simulink subsystem "BatteryMappedSSC"  (R2023a)
settings: Solver=VariableStepAuto  StartTime=0.0  StopTime=10.0  RelTol=1e-3
undefined symbols (not defined in the file): Bat, PlntBattChrgMax, PlntBattIntrnRes, PlntBattNumCellPar, PlntBattNumCellSer, PlntBattOpenCirctVolt, PlntBattSocBpt, PlntBattTempBpt, PlntBattVoltSocBpt
libraries: fl_lib x7, nesl_utility_internal x4, batteryecm_lib x1, nesl_utility x1
settings Model: ModifiedByFormat=The MathWorks, Inc.  Creator=The MathWorks, Inc.  LastModifiedBy=The MathWorks, Inc.
settings OptimizationCC: ReuseModelBlockBuffer=off

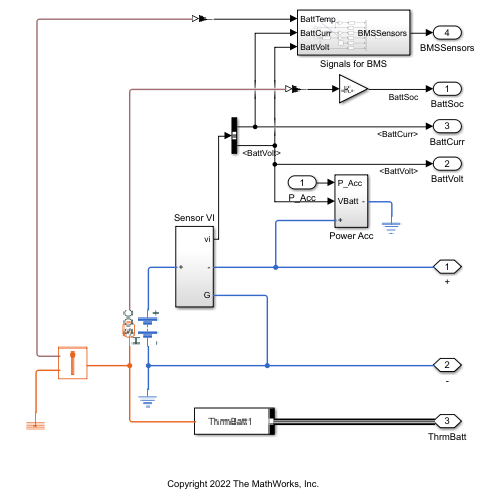
[thumbnail: Simulink's stored preview of the top-level diagram]
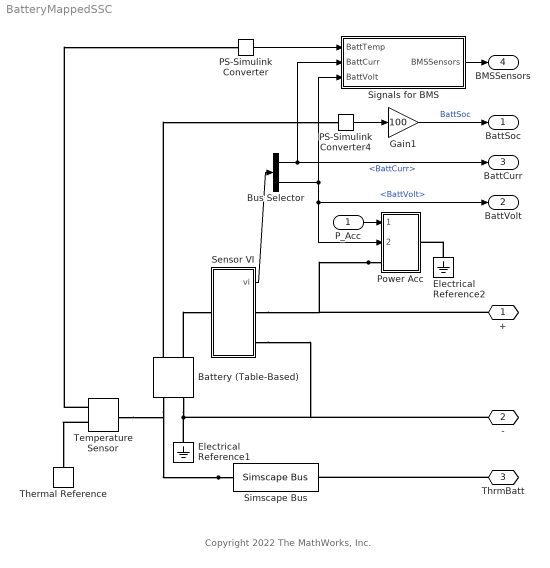
== system BatteryMappedSSC ==
  note: Copyright 2022 The MathWorks, Inc.
  P_Acc : Inport
  Battery (Table-Based) : batteryecm_lib/Battery (Table-Based)  SOC_vec=PlntBattSocBpt  T_dependence=simscape.enum.tablebattery.temperature_dependence.yes  prm_dir=simscape.enum.tablebattery.prm_dir.noCurrentDirectionality  T_vec=PlntBattTempBpt K  V0_mat=repmat(interp1(PlntBattVoltSocBpt, PlntBattOpenCirctVolt, PlntBattSocBpt)', 1, length(PlntBattTempBpt)).*PlntBattNumCellSer V  V0_vec=[3.5057, 3.566, 3.6337, 3.7127, 3.9259, 4.0777, 4.1928] V  V_range=[min(PlntBattOpenCirctVolt), inf].*PlntBattNumCellSer V  R0_mat=PlntBattIntrnRes'.*(PlntBattNumCellSer/PlntBattNumCellPar) Ohm  R0_vec=[.0085, .0085, .0087, .0082, .0083, .0085, .0085] Ohm  R0_dis_mat=[.0117, .0085, .009; .011, .0085, .009; .0114, .0087, .0092; .0107, .0082, .0088; .0107, .0083, .0091; .0113, .0085, .0089; .0116, .0085, .0089] Ohm  R0_dis_vec=[.0085, .0085, .0087, .0082, .0083, .0085, .0085] Ohm  R0_ch_mat=[.0117, .0085, .009; .011, .0085, .009; .0114, .0087, .0092; .0107, .0082, .0088; .0107, .0083, .0091; .0113, .0085, .0089; .0116, .0085, .0089] Ohm  R0_ch_vec=[.0085, .0085, .0087, .0082, .0083, .0085, .0085] Ohm  AH=PlntBattChrgMax*PlntBattNumCellPar A*hr  prm_leak=simscape.enum.tablebattery.prm_leak.disabled  Rleak_vec=[8000, 7000, 6000] Ohm  Rleak=7e3 Ohm  extrapolation_option=simscape.enum.extrapolation.nearest  SOC_port=simscape.enum.tablebattery.enable.yes  prm_dyn=simscape.enum.tablebattery.prm_dyn.off  R1_mat=[.0109, .0029, .0013; .0069, .0024, .0012; .0047, .0026, .0013; .0034, .0016, .001; .0033, .0023, .0014; .0033, .0018, .0011; .0028, .0017, .0011] Ohm  R1_vec=[.0029, .0024, .0026, .0016, .0023, .0018, .0017] Ohm  tau1_mat=[20, 36, 39; 31, 45, 39; 109, 105, 61; 36, 29, 26; 59, 77, 67; 40, 33, 29; 25, 39, 33] s  tau1_vec=[36, 45, 105, 29, 77, 33, 39] s  R2_mat=[.0109, .0029, .0013; .0069, .0024, .0012; .0047, .0026, .0013; .0034, .0016, .001; .0033, .0023, .0014; .0033, .0018, .0011; .0028, .0017, .0011] Ohm  R2_vec=[.0029, .0024, .0026, .0016, .0023, .0018, .0017] Ohm  tau2_mat=[20, 36, 39; 31, 45, 39; 109, 105, 61; 36, 29, 26; 59, 77, 67; 40, 33, 29; 25, 39, 33] s  tau2_vec=[36, 45, 105, 29, 77, 33, 39] s  R3_mat=[.0109, .0029, .0013; .0069, .0024, .0012; .0047, .0026, .0013; .0034, .0016, .001; .0033, .0023, .0014; .0033, .0018, .0011; .0028, .0017, .0011] Ohm  R3_vec=[.0029, .0024, .0026, .0016, .0023, .0018, .0017] Ohm  tau3_mat=[20, 36, 39; 31, 45, 39; 109, 105, 61; 36, 29, 26; 59, 77, 67; 40, 33, 29; 25, 39, 33] s  tau3_vec=[36, 45, 105, 29, 77, 33, 39] s  R4_mat=[.0109, .0029, .0013; .0069, .0024, .0012; .0047, .0026, .0013; .0034, .0016, .001; .0033, .0023, .0014; .0033, .0018, .0011; .0028, .0017, .0011] Ohm  R4_vec=[.0029, .0024, .0026, .0016, .0023, .0018, .0017] Ohm  tau4_mat=[20, 36, 39; 31, 45, 39; 109, 105, 61; 36, 29, 26; 59, 77, 67; 40, 33, 29; 25, 39, 33] s  tau4_vec=[36, 45, 105, 29, 77, 33, 39] s  R5_mat=[.0109, .0029, .0013; .0069, .0024, .0012; .0047, .0026, .0013; .0034, .0016, .001; .0033, .0023, .0014; .0033, .0018, .0011; .0028, .0017, .0011] Ohm  R5_vec=[.0029, .0024, .0026, .0016, .0023, .0018, .0017] Ohm  tau5_mat=[20, 36, 39; 31, 45, 39; 109, 105, 61; 36, 29, 26; 59, 77, 67; 40, 33, 29; 25, 39, 33] s  tau5_vec=[36, 45, 105, 29, 77, 33, 39] s  prm_fade=simscape.enum.tablebattery.prm_fade.disabled  N0=100  dV0=0  dR0=0  dAH=0  dRleak=0  dR1=0  dR2=0  dR3=0  dR4=0  dR5=0  N0vec=[100, 200, 300]  Tfadevec=[298.15, 323.15] K  dV0vec=[0, 0, 0]  dR0vec=[0, 0, 0]  dAHvec=[0, 0, 0]  dRleakvec=[0, 0, 0]  dR1vec=[0, 0, 0]  dR2vec=[0, 0, 0]  dR3vec=[0, 0, 0]  dR4vec=[0, 0, 0]  dR5vec=[0, 0, 0]  dV0mat=[0, 0; 0, 0; 0, 0]  dR0mat=[0, 0; 0, 0; 0, 0]  dAHmat=[0, 0; 0, 0; 0, 0]  dRleakmat=[0, 0; 0, 0; 0, 0]  dR1mat=[0, 0; 0, 0; 0, 0]  dR2mat=[0, 0; 0, 0; 0, 0]  dR3mat=[0, 0; 0, 0; 0, 0]  dR4mat=[0, 0; 0, 0; 0, 0]  dR5mat=[0, 0; 0, 0; 0, 0]  prm_age_modeling=simscape.enum.tablebattery.prm_age_modeling.equation  storage_dt_age_vec=[0] d  storage_T_age_vec=[273] K  prm_age_OCV=simscape.enum.tablebattery.prm_age_OCV.OCV  OCV_age=0.9  SOC_age=0.6  prm_age_resistance=simscape.enum.tablebattery.prm_age.disabled  OCV_scaling_age_resistance=2.2134e6  OCV_offset_age_resistance=1.632e6  temp_exp_age_resistance=0.515833569 V  t_exp_age_resistance=0.75  T_age_vec_resistance=[273.15, 298.15, 323.15] K  dt_age_vec_resistance=[90, 180, 270, 360] d  dR0_age_vec=[0, 0, 0]  t_meas_dR0_age=100 d  dR0_age_mat=[0, 0, 0; 0, 0, 0; 0, 0, 0; 0, 0, 0]  prm_age_capacity=simscape.enum.tablebattery.prm_age.disabled  OCV_scaling_age_capacity=1.5097e07  OCV_offset_age_capacity=8.3625e06  temp_exp_age_capacity=0.6011 V  t_exp_age_capacity=0.75  T_age_vec_capacity=[273.15, 298.15, 323.15] K  dt_age_vec_capacity=[90, 180, 270, 360] d  dAH_age_vec=[0, 0, 0]  t_meas_dAH_age=100 d  dAH_age_mat=[0, 0, 0; 0, 0, 0; 0, 0, 0; 0, 0, 0]  thermal_port=simscape.enum.thermaleffects.model  temperature=298.15 K  thermal_mass=PlntDCDCThermMass*PlntBattNumCellSer*PlntBattModNumCellPar % Parameter assumed J/K  i_specify=off  i_priority=None  i=0 A  i_nominal_specify=off  i_nominal_unit=A  i_nominal_value=1  v_specify=off  v_priority=None  v=0 V  v_nominal_specify=off  v_nominal_unit=V  v_nominal_value=1  stateOfCharge_specify=on  stateOfCharge_priority=High  stateOfCharge=PlntBattSocInit  stateOfCharge_nominal_specify=off  stateOfCharge_nominal_unit=1  stateOfCharge_nominal_value=1  num_cycles_specify=off  num_cycles_priority=High  num_cycles=0  num_cycles_nominal_specify=off  num_cycles_nominal_unit=1  num_cycles_nominal_value=1  cell_temperature_specify=on  cell_temperature_priority=High  cell_temperature=PlntBattTempInitDegC degC  cell_temperature_nominal_specify=off  cell_temperature_nominal_unit=K  cell_temperature_nominal_value=1
  Bus Selector : BusSelector  OutputSignals=BattCurr,BattVolt
  Electrical Reference1 : fl_lib/Electrical/Electrical Elements/Electrical Reference
  Electrical Reference2 : fl_lib/Electrical/Electrical Elements/Electrical Reference
  Gain1 : Gain  Gain=100
  PS-Simulink Converter : nesl_utility/PS-Simulink Converter  PhysicalDomain=network_engine_domain  SubClassName=ps_output  LeftPortType=input  RightPortType=output  PseudoPeriodic=off  Frequencies=[]  VectorFormat=inherit  Unit=inherit  AffineConversion=off
  PS-Simulink Converter4 : nesl_utility_internal/PS-Simulink Converter  PhysicalDomain=network_engine_domain  SubClassName=ps_output  LeftPortType=input  RightPortType=output  PseudoPeriodic=off  Frequencies=[]  VectorFormat=1-D array  Unit=1  AffineConversion=off
  Power Acc : Subsystem
  Sensor VI : Subsystem
  Signals for BMS : Subsystem
  Simscape Bus : SimscapeBus  HierarchyStrings=ThrmBatt1
  Temperature Sensor : fl_lib/Thermal/Thermal Sensors/Temperature Sensor  temperature_measure=foundation.enum.MeasurementReference.difference
  Thermal Reference : fl_lib/Thermal/Thermal Elements/Thermal Reference
  + : PMIOPort  Side=Right
  - : PMIOPort  Port=2  Side=Right
  ThrmBatt : PMIOPort  Port=3  Side=Right
  BattSoc : Outport
  BattVolt : Outport  Port=2
  BattCurr : Outport  Port=3
  BMSSensors : Outport  Port=4  VectorParamsAs1DForOutWhenUnconnected=off
  wires:
  PS-Simulink Converter4/1 -> Gain1/1
  Bus Selector/1 -> Signals for BMS/2(BattCurr), BattCurr/1  "<BattCurr>"
  Sensor VI/1(vi) -> Bus Selector/1
  Gain1/1 -> BattSoc/1  "BattSoc"
  Bus Selector/2 -> Signals for BMS/3(BattVolt), Power Acc/2(VBatt), BattVolt/1  "<BattVolt>"
  P_Acc/1 -> Power Acc/1(P_Acc)
  Signals for BMS/1(BMSSensors) -> BMSSensors/1
  PS-Simulink Converter/1 -> Signals for BMS/1(BattTemp)
  connections:
  Battery (Table-Based)/RConn1 -- Sensor VI/RConn2 -- -/RConn1 -- Electrical Reference1/LConn1
  Power Acc/LConn1 -- Sensor VI/RConn1 -- +/RConn1
  Simscape Bus/LConn1 -- Temperature Sensor/LConn1 -- Battery (Table-Based)/RConn2
  Battery (Table-Based)/LConn1 -- Sensor VI/LConn1
  Electrical Reference2/LConn1 -- Power Acc/RConn1
  Battery (Table-Based)/LConn2 -- PS-Simulink Converter4/LConn1
  Temperature Sensor/RConn1 -- Thermal Reference/LConn1
  Temperature Sensor/RConn2 -- PS-Simulink Converter/LConn1
  ThrmBatt/RConn1 -- Simscape Bus/RConn1

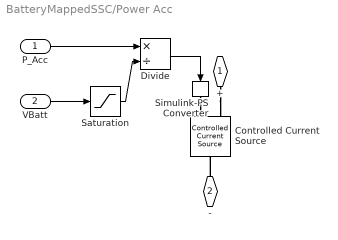
== system BatteryMappedSSC/Power Acc ==
  P_Acc : Inport
  VBatt : Inport  Port=2
  Controlled Current Source : fl_lib/Electrical/Electrical Sources/Controlled Current Source
  Divide : Product  Inputs=*/
  Saturation : Saturate  UpperLimit=inf  LowerLimit=min(Bat.noLoadV, [], 'all')  ZeroCross=off
  Simulink-PS Converter : nesl_utility_internal/Simulink-PS Converter  PhysicalDomain=network_engine_domain  SubClassName=ps_input  LeftPortType=input  RightPortType=output  PseudoPeriodic=off  Frequencies=[]  NoiseDistribution=none  NoiseParameters=[]  Unit=A  AffineConversion=off  FilteringAndDerivatives=filter  SimscapeFilterOrder=1  InputFilterTimeConstant=0.001  UdotUserProvided=0
  + : PMIOPort  Side=Left
  - : PMIOPort  Port=2  Side=Right
  wires:
  VBatt/1 -> Saturation/1
  P_Acc/1 -> Divide/1
  Divide/1 -> Simulink-PS Converter/1
  Saturation/1 -> Divide/2
  connections:
  -/RConn1 -- Controlled Current Source/LConn1
  +/RConn1 -- Controlled Current Source/RConn2
  Simulink-PS Converter/RConn1 -- Controlled Current Source/RConn1

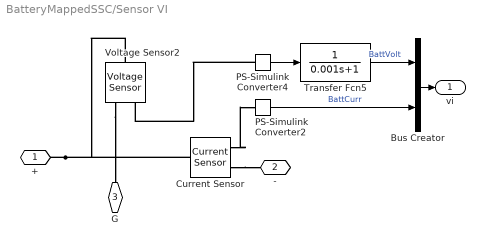
== system BatteryMappedSSC/Sensor VI ==
  Bus Creator : BusCreator  Inputs=2
  Current Sensor : fl_lib/Electrical/Electrical Sensors/Current Sensor
  PS-Simulink Converter2 : nesl_utility_internal/PS-Simulink Converter  PhysicalDomain=network_engine_domain  SubClassName=ps_output  LeftPortType=input  RightPortType=output  PseudoPeriodic=off  Frequencies=[]  VectorFormat=1-D array  Unit=1  AffineConversion=off
  PS-Simulink Converter4 : nesl_utility_internal/PS-Simulink Converter  PhysicalDomain=network_engine_domain  SubClassName=ps_output  LeftPortType=input  RightPortType=output  PseudoPeriodic=off  Frequencies=[]  VectorFormat=1-D array  Unit=1  AffineConversion=off
  Transfer Fcn5 : TransferFcn  Denominator=[0.001 1]
  Voltage Sensor2 : fl_lib/Electrical/Electrical Sensors/Voltage Sensor
  + : PMIOPort  Side=Left
  - : PMIOPort  Port=2  Side=Right
  G : PMIOPort  Port=3  Side=Right
  vi : Outport
  wires:
  Transfer Fcn5/1 -> Bus Creator/1  "BattVolt"
  PS-Simulink Converter2/1 -> Bus Creator/2  "BattCurr"
  PS-Simulink Converter4/1 -> Transfer Fcn5/1
  Bus Creator/1 -> vi/1
  connections:
  +/RConn1 -- Current Sensor/LConn1 -- Voltage Sensor2/LConn1
  PS-Simulink Converter4/LConn1 -- Voltage Sensor2/RConn1
  Current Sensor/RConn2 -- -/RConn1
  Voltage Sensor2/RConn2 -- G/RConn1
  Current Sensor/RConn1 -- PS-Simulink Converter2/LConn1

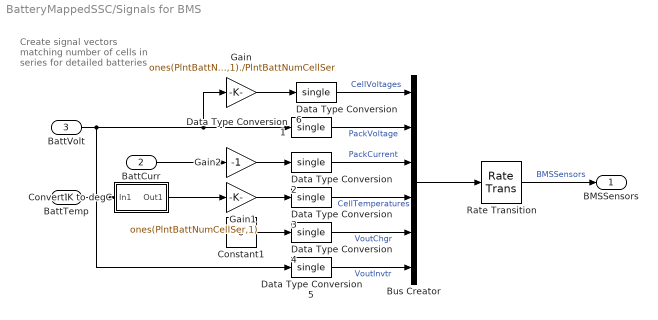
== system BatteryMappedSSC/Signals for BMS ==
  note: Create signal vectors
      | matching number of
      | cells in series for
      | detailed batteries
  BattTemp : Inport
  BattCurr : Inport  Port=2
  BattVolt : Inport  Port=3
  Bus Creator : BusCreator  Inputs=6
  Constant1 : Constant  Value=0
  Convert K to degC : Subsystem
  Data Type Conversion{1..6} (6 alike) : DataTypeConversion  OutDataTypeStr=single  SaturateOnIntegerOverflow=off  RndMeth=Floor
  Gain : Gain  Gain=ones(PlntBattNumCellSer,1)./PlntBattNumCellSer
  Gain1 : Gain  Gain=ones(PlntBattNumCellSer,1)
  Gain2 : Gain  Gain=-1
  Rate Transition : RateTransition  OutPortSampleTime=0.1
  BMSSensors : Outport
  wires:
  BattCurr/1 -> Gain2/1
  Constant1/1 -> Data Type Conversion4/1
  BattVolt/1 -> Data Type Conversion1/1, Gain/1, Data Type Conversion5/1
  Gain/1 -> Data Type Conversion6/1
  BattTemp/1 -> Convert K to degC/1(In1)
  Data Type Conversion4/1 -> Bus Creator/5  "VoutChgr"
  Gain1/1 -> Data Type Conversion3/1
  Data Type Conversion5/1 -> Bus Creator/6  "VoutInvtr"
  Gain2/1 -> Data Type Conversion2/1
  Convert K to degC/1(Out1) -> Gain1/1
  Bus Creator/1 -> Rate Transition/1
  Data Type Conversion1/1 -> Bus Creator/2  "PackVoltage"
  Data Type Conversion6/1 -> Bus Creator/1  "CellVoltages"
  Data Type Conversion2/1 -> Bus Creator/3  "PackCurrent"
  Data Type Conversion3/1 -> Bus Creator/4  "CellTemperatures"
  Rate Transition/1 -> BMSSensors/1  "BMSSensors"

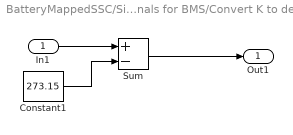
== system BatteryMappedSSC/Signals for BMS/Convert K to degC ==
  In1 : Inport
  Constant1 : Constant  Value=273.15
  Sum : Sum  Inputs=+-
  Out1 : Outport
  wires:
  Sum/1 -> Out1/1
  Constant1/1 -> Sum/2
  In1/1 -> Sum/1
